simulink model "ex_4"  (R2016a)
settings: Solver=VariableStepAuto  StartTime=0.0  StopTime=10.0  RelTol=1e-3
settings Model: Creator=Linstar  LastModifiedBy=Linstar

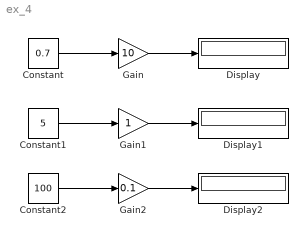
== system ex_4 ==
  Constant : Constant  Value=0.7
  Constant1 : Constant  Value=5
  Constant2 : Constant  Value=100
  Display : Display
  Display1 : Display
  Display2 : Display
  Gain : Gain  Gain=10
  Gain1 : Gain
  Gain2 : Gain  Gain=0.1
  wires:
  Constant/1 -> Gain/1
  Gain/1 -> Display/1
  Constant1/1 -> Gain1/1
  Gain1/1 -> Display1/1
  Constant2/1 -> Gain2/1
  Gain2/1 -> Display2/1
